simulink model "MLH2025"  (R2024b)
settings: Solver=VariableStepAuto  StartTime=0.0  StopTime=10.0  RelTol=1e-3
undefined symbols (not defined in the file): B, MPLX, Pi, PWM
settings Model: Creator=el2jo  LastModifiedBy=el2jo

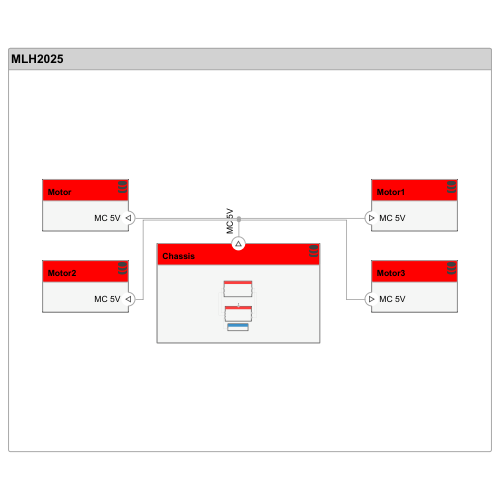
[thumbnail: Simulink's stored preview of the top-level diagram]
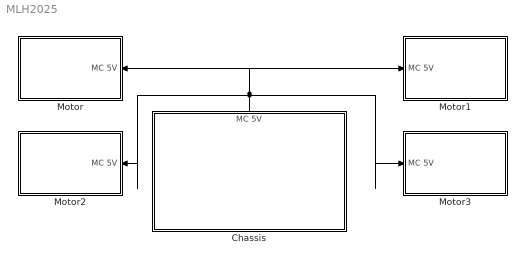
== system MLH2025 ==
  "Chassis " : Subsystem
      settings: PortSchema="{\"entries\":[{\"content\":{\"headerSize\":26,\"margin\":15,\"minimumSpacing\":25,\"sides\":[{\"content\":{},\"type\":\"ConnectorPlacement.EquallySpacedRectSide\",\"uuid\":\"9dc2c90c-aec4-43c7-8746-b592e26bfa16\"},{\"content\":{\"side\":\"RIGHT\"},\"type\":\"ConnectorPlacement.EquallySpacedRectSide\",\"uuid\":\"bdfb89bc-8823-48a4-99ae-46e8d46d5f72\"},{\"content\":{\"connectorIds\":[\"Out1\"],\"side\":\"TOP\"},\"type\":\"ConnectorPlacement.EquallySpacedRectSide\",\"uuid\":\"226bc484-5c65-4ece-8f5d-0589859e3e31\"}]},\"type\":\"ConnectorPlacement.EquallySpacedConnector\",\"uuid\":\"f9cc3cfe-bad8-451a-a9a4-a5a609f97b74\"}],\"packageUris\":[\"http://schema.mathworks.com/mf0/Connector/R2020b\"],\"version\":\"1.0\"}"
  Motor : Subsystem
      settings: PortSchema="{\"entries\":[{\"content\":{\"headerSize\":26,\"margin\":15,\"minimumSpacing\":25,\"sides\":[{\"content\":{},\"type\":\"ConnectorPlacement.EquallySpacedRectSide\",\"uuid\":\"9dc2c90c-aec4-43c7-8746-b592e26bfa16\"},{\"content\":{\"connectorIds\":[\"In1\"],\"side\":\"RIGHT\"},\"type\":\"ConnectorPlacement.EquallySpacedRectSide\",\"uuid\":\"bdfb89bc-8823-48a4-99ae-46e8d46d5f72\"},{\"content\":{\"side\":\"TOP\"},\"type\":\"ConnectorPlacement.EquallySpacedRectSide\",\"uuid\":\"226bc484-5c65-4ece-8f5d-0589859e3e31\"}]},\"type\":\"ConnectorPlacement.EquallySpacedConnector\",\"uuid\":\"f9cc3cfe-bad8-451a-a9a4-a5a609f97b74\"}],\"packageUris\":[\"http://schema.mathworks.com/mf0/Connector/R2020b\"],\"version\":\"1.0\"}"
  Motor1 : Subsystem
      settings: PortSchema="{\"entries\":[{\"content\":{\"headerSize\":26,\"margin\":15,\"minimumSpacing\":25,\"sides\":[{\"content\":{\"connectorIds\":[\"In1\"]},\"type\":\"ConnectorPlacement.EquallySpacedRectSide\",\"uuid\":\"9dc2c90c-aec4-43c7-8746-b592e26bfa16\"},{\"content\":{\"side\":\"RIGHT\"},\"type\":\"ConnectorPlacement.EquallySpacedRectSide\",\"uuid\":\"bdfb89bc-8823-48a4-99ae-46e8d46d5f72\"},{\"content\":{\"side\":\"TOP\"},\"type\":\"ConnectorPlacement.EquallySpacedRectSide\",\"uuid\":\"226bc484-5c65-4ece-8f5d-0589859e3e31\"}]},\"type\":\"ConnectorPlacement.EquallySpacedConnector\",\"uuid\":\"f9cc3cfe-bad8-451a-a9a4-a5a609f97b74\"}],\"packageUris\":[\"http://schema.mathworks.com/mf0/Connector/R2020b\"],\"version\":\"1.0\"}"
  Motor2 : Subsystem
      settings: PortSchema="{\"entries\":[{\"content\":{\"headerSize\":26,\"margin\":15,\"minimumSpacing\":25,\"sides\":[{\"content\":{},\"type\":\"ConnectorPlacement.EquallySpacedRectSide\",\"uuid\":\"9dc2c90c-aec4-43c7-8746-b592e26bfa16\"},{\"content\":{\"connectorIds\":[\"In1\"],\"side\":\"RIGHT\"},\"type\":\"ConnectorPlacement.EquallySpacedRectSide\",\"uuid\":\"bdfb89bc-8823-48a4-99ae-46e8d46d5f72\"},{\"content\":{\"side\":\"TOP\"},\"type\":\"ConnectorPlacement.EquallySpacedRectSide\",\"uuid\":\"226bc484-5c65-4ece-8f5d-0589859e3e31\"}]},\"type\":\"ConnectorPlacement.EquallySpacedConnector\",\"uuid\":\"f9cc3cfe-bad8-451a-a9a4-a5a609f97b74\"}],\"packageUris\":[\"http://schema.mathworks.com/mf0/Connector/R2020b\"],\"version\":\"1.0\"}"
  Motor3 : Subsystem
      settings: PortSchema="{\"entries\":[{\"content\":{\"headerSize\":26,\"margin\":15,\"minimumSpacing\":25,\"sides\":[{\"content\":{\"connectorIds\":[\"In1\"]},\"type\":\"ConnectorPlacement.EquallySpacedRectSide\",\"uuid\":\"9dc2c90c-aec4-43c7-8746-b592e26bfa16\"},{\"content\":{\"side\":\"RIGHT\"},\"type\":\"ConnectorPlacement.EquallySpacedRectSide\",\"uuid\":\"bdfb89bc-8823-48a4-99ae-46e8d46d5f72\"},{\"content\":{\"side\":\"TOP\"},\"type\":\"ConnectorPlacement.EquallySpacedRectSide\",\"uuid\":\"226bc484-5c65-4ece-8f5d-0589859e3e31\"}]},\"type\":\"ConnectorPlacement.EquallySpacedConnector\",\"uuid\":\"f9cc3cfe-bad8-451a-a9a4-a5a609f97b74\"}],\"packageUris\":[\"http://schema.mathworks.com/mf0/Connector/R2020b\"],\"version\":\"1.0\"}"
  wires:
  "Chassis "/1(MC 5V) -> Motor/1(MC 5V), Motor1/1(MC 5V), Motor3/1(MC 5V), Motor2/1(MC 5V)

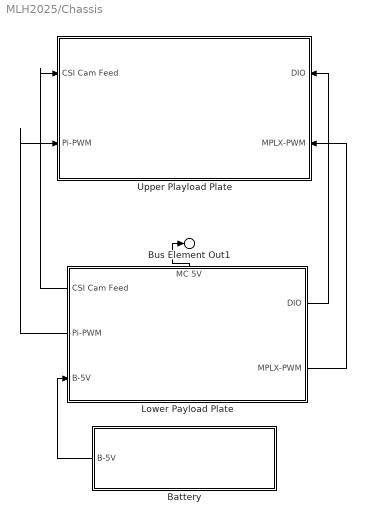
== system MLH2025/Chassis  ==
  Battery : Subsystem
      settings: PortSchema="{\"entries\":[{\"content\":{\"headerSize\":26,\"margin\":15,\"minimumSpacing\":25,\"sides\":[{\"content\":{\"connectorIds\":[\"Out1\"]},\"type\":\"ConnectorPlacement.EquallySpacedRectSide\",\"uuid\":\"9dc2c90c-aec4-43c7-8746-b592e26bfa16\"},{\"content\":{\"side\":\"RIGHT\"},\"type\":\"ConnectorPlacement.EquallySpacedRectSide\",\"uuid\":\"bdfb89bc-8823-48a4-99ae-46e8d46d5f72\"},{\"content\":{\"side\":\"TOP\"},\"type\":\"ConnectorPlacement.EquallySpacedRectSide\",\"uuid\":\"226bc484-5c65-4ece-8f5d-0589859e3e31\"}]},\"type\":\"ConnectorPlacement.EquallySpacedConnector\",\"uuid\":\"f9cc3cfe-bad8-451a-a9a4-a5a609f97b74\"}],\"packageUris\":[\"http://schema.mathworks.com/mf0/Connector/R2020b\"],\"version\":\"1.0\"}"
  Lower Payload Plate : Subsystem
      settings: PortSchema="{\"entries\":[{\"content\":{\"headerSize\":26,\"margin\":15,\"minimumSpacing\":25,\"sides\":[{\"content\":{\"connectorIds\":[\"Out1\",\"Out4\",\"In1\"]},\"type\":\"ConnectorPlacement.EquallySpacedRectSide\",\"uuid\":\"9dc2c90c-aec4-43c7-8746-b592e26bfa16\"},{\"content\":{\"connectorIds\":[\"Out3\",\"Out5\"],\"side\":\"RIGHT\"},\"type\":\"ConnectorPlacement.EquallySpacedRectSide\",\"uuid\":\"bdfb89bc-8823-48a4-99ae-46e8d46d5f72\"},{\"content\":{\"connectorIds\":[\"Out2\"],\"side\":\"TOP\"},\"type\":\"ConnectorPlacement.EquallySpacedRectSide\",\"uuid\":\"226bc484-5c65-4ece-8f5d-0589859e3e31\"}]},\"type\":\"ConnectorPlacement.EquallySpacedConnector\",\"uuid\":\"f9cc3cfe-bad8-451a-a9a4-a5a609f97b74\"}],\"packageUris\":[\"http://schema.mathworks.com/mf0/Connector/R2020b\"],\"version\":\"1.0\"}"
  Upper Playload Plate : Subsystem
      settings: PortSchema="{\"entries\":[{\"content\":{\"headerSize\":26,\"margin\":15,\"minimumSpacing\":25,\"sides\":[{\"content\":{\"connectorIds\":[\"In1\",\"In3\"]},\"type\":\"ConnectorPlacement.EquallySpacedRectSide\",\"uuid\":\"9dc2c90c-aec4-43c7-8746-b592e26bfa16\"},{\"content\":{\"connectorIds\":[\"In2\",\"In4\"],\"side\":\"RIGHT\"},\"type\":\"ConnectorPlacement.EquallySpacedRectSide\",\"uuid\":\"bdfb89bc-8823-48a4-99ae-46e8d46d5f72\"},{\"content\":{\"side\":\"TOP\"},\"type\":\"ConnectorPlacement.EquallySpacedRectSide\",\"uuid\":\"226bc484-5c65-4ece-8f5d-0589859e3e31\"}]},\"type\":\"ConnectorPlacement.EquallySpacedConnector\",\"uuid\":\"f9cc3cfe-bad8-451a-a9a4-a5a609f97b74\"}],\"packageUris\":[\"http://schema.mathworks.com/mf0/Connector/R2020b\"],\"version\":\"1.0\"}"
  Bus Element Out1 : Outport  PortName=MC 5V
  wires:
  Lower Payload Plate/5(MPLX-PWM) -> Upper Playload Plate/4(MPLX-PWM)
  Lower Payload Plate/4(Pi-PWM) -> Upper Playload Plate/3(Pi-PWM)
  Lower Payload Plate/3(DIO) -> Upper Playload Plate/2(DIO)
  Battery/1(B-5V) -> Lower Payload Plate/1(B-5V)
  Lower Payload Plate/2(MC 5V) -> Bus Element Out1/1
  Lower Payload Plate/1(CSI Cam Feed) -> Upper Playload Plate/1(CSI Cam Feed)

== system MLH2025/Motor ==
  Bus Element In1 : Inport  PortName=MC 5V

== system MLH2025/Motor1 ==
  Bus Element In1 : Inport  PortName=MC 5V

== system MLH2025/Motor2 ==
  Bus Element In1 : Inport  PortName=MC 5V

== system MLH2025/Motor3 ==
  Bus Element In1 : Inport  PortName=MC 5V

== system MLH2025/Chassis /Battery ==
  Bus Element Out1 : Outport  PortName=B-5V

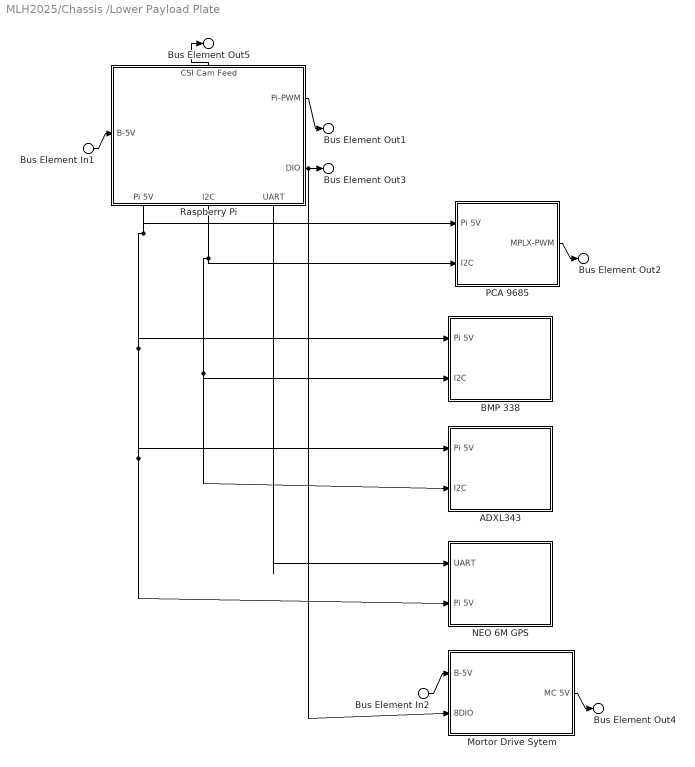
== system MLH2025/Chassis /Lower Payload Plate ==
  Bus Element In1 : Inport  PortName=B-5V
  Bus Element In2 : Inport  PortName=B-5V
  ADXL343 : Subsystem
      settings: PortSchema="{\"entries\":[{\"content\":{\"headerSize\":26,\"margin\":15,\"minimumSpacing\":25,\"sides\":[{\"content\":{\"connectorIds\":[\"In1\",\"In2\"]},\"type\":\"ConnectorPlacement.EquallySpacedRectSide\",\"uuid\":\"9dc2c90c-aec4-43c7-8746-b592e26bfa16\"},{\"content\":{\"side\":\"RIGHT\"},\"type\":\"ConnectorPlacement.EquallySpacedRectSide\",\"uuid\":\"bdfb89bc-8823-48a4-99ae-46e8d46d5f72\"},{\"content\":{\"side\":\"TOP\"},\"type\":\"ConnectorPlacement.EquallySpacedRectSide\",\"uuid\":\"226bc484-5c65-4ece-8f5d-0589859e3e31\"}]},\"type\":\"ConnectorPlacement.EquallySpacedConnector\",\"uuid\":\"f9cc3cfe-bad8-451a-a9a4-a5a609f97b74\"}],\"packageUris\":[\"http://schema.mathworks.com/mf0/Connector/R2020b\"],\"version\":\"1.0\"}"
  BMP 338 : Subsystem
      settings: PortSchema="{\"entries\":[{\"content\":{\"headerSize\":26,\"margin\":15,\"minimumSpacing\":25,\"sides\":[{\"content\":{\"connectorIds\":[\"In1\",\"In2\"]},\"type\":\"ConnectorPlacement.EquallySpacedRectSide\",\"uuid\":\"9dc2c90c-aec4-43c7-8746-b592e26bfa16\"},{\"content\":{\"side\":\"RIGHT\"},\"type\":\"ConnectorPlacement.EquallySpacedRectSide\",\"uuid\":\"bdfb89bc-8823-48a4-99ae-46e8d46d5f72\"},{\"content\":{\"side\":\"TOP\"},\"type\":\"ConnectorPlacement.EquallySpacedRectSide\",\"uuid\":\"226bc484-5c65-4ece-8f5d-0589859e3e31\"},{\"content\":{\"side\":\"BOTTOM\"},\"type\":\"ConnectorPlacement.EquallySpacedRectSide\",\"uuid\":\"99e16435-73fc-4f11-a495-18abe58af7ce\"}]},\"type\":\"ConnectorPlacement.EquallySpacedConnector\",\"uuid\":\"f9cc3cfe-bad8-451a-a9a4-a5a609f97b74\"}],\"packageUris\":[\"http://schema.mathworks.com/mf0/Connector/R2020b\"],\"version\":\"1.0\"}"
  Mortor Drive Sytem : Subsystem
      settings: PortSchema="{\"entries\":[{\"content\":{\"headerSize\":26,\"margin\":15,\"minimumSpacing\":25,\"sides\":[{\"content\":{\"connectorIds\":[\"In1\",\"In2\"]},\"type\":\"ConnectorPlacement.EquallySpacedRectSide\",\"uuid\":\"9dc2c90c-aec4-43c7-8746-b592e26bfa16\"},{\"content\":{\"connectorIds\":[\"Out1\"],\"side\":\"RIGHT\"},\"type\":\"ConnectorPlacement.EquallySpacedRectSide\",\"uuid\":\"bdfb89bc-8823-48a4-99ae-46e8d46d5f72\"},{\"content\":{\"side\":\"TOP\"},\"type\":\"ConnectorPlacement.EquallySpacedRectSide\",\"uuid\":\"226bc484-5c65-4ece-8f5d-0589859e3e31\"},{\"content\":{\"side\":\"BOTTOM\"},\"type\":\"ConnectorPlacement.EquallySpacedRectSide\",\"uuid\":\"135a2d99-9543-48c1-84f1-a8adb7010785\"}]},\"type\":\"ConnectorPlacement.EquallySpacedConnector\",\"uuid\":\"f9cc3cfe-bad8-451a-a9a4-a5a609f97b74\"}],\"packageUris\":[\"http://schema.mathworks.com/mf0/Connector/R2020b\"],\"version\":\"1.0\"}"
  NEO 6M GPS : Subsystem
      settings: PortSchema="{\"entries\":[{\"content\":{\"headerSize\":26,\"margin\":15,\"minimumSpacing\":25,\"sides\":[{\"content\":{\"connectorIds\":[\"In2\",\"In1\"]},\"type\":\"ConnectorPlacement.EquallySpacedRectSide\",\"uuid\":\"9dc2c90c-aec4-43c7-8746-b592e26bfa16\"},{\"content\":{\"side\":\"RIGHT\"},\"type\":\"ConnectorPlacement.EquallySpacedRectSide\",\"uuid\":\"bdfb89bc-8823-48a4-99ae-46e8d46d5f72\"},{\"content\":{\"side\":\"TOP\"},\"type\":\"ConnectorPlacement.EquallySpacedRectSide\",\"uuid\":\"226bc484-5c65-4ece-8f5d-0589859e3e31\"},{\"content\":{\"side\":\"BOTTOM\"},\"type\":\"ConnectorPlacement.EquallySpacedRectSide\",\"uuid\":\"07c50740-44ff-450e-bd99-694483ad2c77\"}]},\"type\":\"ConnectorPlacement.EquallySpacedConnector\",\"uuid\":\"f9cc3cfe-bad8-451a-a9a4-a5a609f97b74\"}],\"packageUris\":[\"http://schema.mathworks.com/mf0/Connector/R2020b\"],\"version\":\"1.0\"}"
  PCA 9685 : Subsystem
      settings: PortSchema="{\"entries\":[{\"content\":{\"headerSize\":26,\"margin\":15,\"minimumSpacing\":25,\"sides\":[{\"content\":{\"connectorIds\":[\"In1\",\"In2\"]},\"type\":\"ConnectorPlacement.EquallySpacedRectSide\",\"uuid\":\"9dc2c90c-aec4-43c7-8746-b592e26bfa16\"},{\"content\":{\"connectorIds\":[\"Out1\"],\"side\":\"RIGHT\"},\"type\":\"ConnectorPlacement.EquallySpacedRectSide\",\"uuid\":\"bdfb89bc-8823-48a4-99ae-46e8d46d5f72\"},{\"content\":{\"side\":\"TOP\"},\"type\":\"ConnectorPlacement.EquallySpacedRectSide\",\"uuid\":\"226bc484-5c65-4ece-8f5d-0589859e3e31\"}]},\"type\":\"ConnectorPlacement.EquallySpacedConnector\",\"uuid\":\"f9cc3cfe-bad8-451a-a9a4-a5a609f97b74\"}],\"packageUris\":[\"http://schema.mathworks.com/mf0/Connector/R2020b\"],\"version\":\"1.0\"}"
  "Raspberry Pi " : Subsystem
      settings: PortSchema="{\"entries\":[{\"content\":{\"headerSize\":26,\"margin\":15,\"minimumSpacing\":25,\"sides\":[{\"content\":{\"connectorIds\":[\"In1\"]},\"type\":\"ConnectorPlacement.EquallySpacedRectSide\",\"uuid\":\"9dc2c90c-aec4-43c7-8746-b592e26bfa16\"},{\"content\":{\"connectorIds\":[\"Out2\",\"Out3\"],\"side\":\"RIGHT\"},\"type\":\"ConnectorPlacement.EquallySpacedRectSide\",\"uuid\":\"bdfb89bc-8823-48a4-99ae-46e8d46d5f72\"},{\"content\":{\"connectorIds\":[\"Out1\"],\"side\":\"TOP\"},\"type\":\"ConnectorPlacement.EquallySpacedRectSide\",\"uuid\":\"226bc484-5c65-4ece-8f5d-0589859e3e31\"},{\"content\":{\"connectorIds\":[\"Out4\",\"Out5\",\"Out6\"],\"side\":\"BOTTOM\"},\"type\":\"ConnectorPlacement.EquallySpacedRectSide\",\"uuid\":\"e2d5389b-7d33-4c7a-8f47-39975d75565d\"}]},\"type\":\"ConnectorPlacement.EquallySpacedConnector\",\"uuid\":\"f9cc3cfe-bad8-451a-a9a4-a5a609f97b74\"}],\"packageUris\":[\"http://schema.mathworks.com/mf0/Connector/R2020b\"],\"version\":\"1.0\"}"
  Bus Element Out5 : Outport  PortName=CSI Cam Feed
  Bus Element Out4 : Outport  Port=2  PortName=MC 5V
  Bus Element Out3 : Outport  Port=3  PortName=DIO
  Bus Element Out1 : Outport  Port=4  PortName=Pi-PWM
  Bus Element Out2 : Outport  Port=5  PortName=MPLX-PWM
  wires:
  Bus Element In1/1 -> "Raspberry Pi "/1(B-5V)
  "Raspberry Pi "/2(Pi-PWM) -> Bus Element Out1/1
  "Raspberry Pi "/4("Pi 5V ") -> NEO 6M GPS/1("Pi 5V "), ADXL343/1("Pi 5V "), BMP 338/1("Pi 5V "), PCA 9685/1("Pi 5V ")
  Bus Element In2/1 -> Mortor Drive Sytem/1(B-5V)
  "Raspberry Pi "/5(I2C) -> BMP 338/2(I2C), ADXL343/2(I2C), PCA 9685/2(I2C)
  "Raspberry Pi "/6(UART) -> NEO 6M GPS/2(UART)
  "Raspberry Pi "/3(DIO) -> Mortor Drive Sytem/2(8DIO), Bus Element Out3/1
  "Raspberry Pi "/1(CSI Cam Feed) -> Bus Element Out5/1
  PCA 9685/1(MPLX-PWM) -> Bus Element Out2/1
  Mortor Drive Sytem/1(MC 5V) -> Bus Element Out4/1

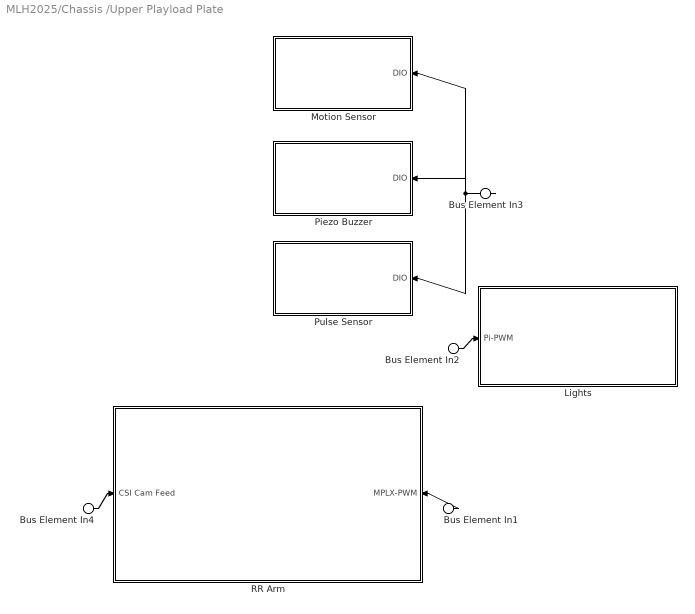
== system MLH2025/Chassis /Upper Playload Plate ==
  Bus Element In4 : Inport  PortName=CSI Cam Feed
  Bus Element In3 : Inport  Port=2  PortName=DIO
  Bus Element In2 : Inport  Port=3  PortName=Pi-PWM
  Bus Element In1 : Inport  Port=4  PortName=MPLX-PWM
  Lights : Subsystem
      settings: PortSchema="{\"entries\":[{\"content\":{\"headerSize\":26,\"margin\":15,\"minimumSpacing\":25,\"sides\":[{\"content\":{\"connectorIds\":[\"In1\"]},\"type\":\"ConnectorPlacement.EquallySpacedRectSide\",\"uuid\":\"9dc2c90c-aec4-43c7-8746-b592e26bfa16\"},{\"content\":{\"side\":\"RIGHT\"},\"type\":\"ConnectorPlacement.EquallySpacedRectSide\",\"uuid\":\"bdfb89bc-8823-48a4-99ae-46e8d46d5f72\"},{\"content\":{\"side\":\"TOP\"},\"type\":\"ConnectorPlacement.EquallySpacedRectSide\",\"uuid\":\"226bc484-5c65-4ece-8f5d-0589859e3e31\"}]},\"type\":\"ConnectorPlacement.EquallySpacedConnector\",\"uuid\":\"f9cc3cfe-bad8-451a-a9a4-a5a609f97b74\"}],\"packageUris\":[\"http://schema.mathworks.com/mf0/Connector/R2020b\"],\"version\":\"1.0\"}"
  Motion Sensor : Subsystem
      settings: PortSchema="{\"entries\":[{\"content\":{\"headerSize\":26,\"margin\":15,\"minimumSpacing\":25,\"sides\":[{\"content\":{},\"type\":\"ConnectorPlacement.EquallySpacedRectSide\",\"uuid\":\"9dc2c90c-aec4-43c7-8746-b592e26bfa16\"},{\"content\":{\"connectorIds\":[\"In1\"],\"side\":\"RIGHT\"},\"type\":\"ConnectorPlacement.EquallySpacedRectSide\",\"uuid\":\"bdfb89bc-8823-48a4-99ae-46e8d46d5f72\"},{\"content\":{\"side\":\"TOP\"},\"type\":\"ConnectorPlacement.EquallySpacedRectSide\",\"uuid\":\"226bc484-5c65-4ece-8f5d-0589859e3e31\"}]},\"type\":\"ConnectorPlacement.EquallySpacedConnector\",\"uuid\":\"f9cc3cfe-bad8-451a-a9a4-a5a609f97b74\"}],\"packageUris\":[\"http://schema.mathworks.com/mf0/Connector/R2020b\"],\"version\":\"1.0\"}"
  Piezo Buzzer : Subsystem
      settings: PortSchema="{\"entries\":[{\"content\":{\"headerSize\":26,\"margin\":15,\"minimumSpacing\":25,\"sides\":[{\"content\":{},\"type\":\"ConnectorPlacement.EquallySpacedRectSide\",\"uuid\":\"9dc2c90c-aec4-43c7-8746-b592e26bfa16\"},{\"content\":{\"connectorIds\":[\"In1\"],\"side\":\"RIGHT\"},\"type\":\"ConnectorPlacement.EquallySpacedRectSide\",\"uuid\":\"bdfb89bc-8823-48a4-99ae-46e8d46d5f72\"},{\"content\":{\"side\":\"TOP\"},\"type\":\"ConnectorPlacement.EquallySpacedRectSide\",\"uuid\":\"226bc484-5c65-4ece-8f5d-0589859e3e31\"}]},\"type\":\"ConnectorPlacement.EquallySpacedConnector\",\"uuid\":\"f9cc3cfe-bad8-451a-a9a4-a5a609f97b74\"}],\"packageUris\":[\"http://schema.mathworks.com/mf0/Connector/R2020b\"],\"version\":\"1.0\"}"
  Pulse Sensor : Subsystem
      settings: PortSchema="{\"entries\":[{\"content\":{\"headerSize\":26,\"margin\":15,\"minimumSpacing\":25,\"sides\":[{\"content\":{},\"type\":\"ConnectorPlacement.EquallySpacedRectSide\",\"uuid\":\"9dc2c90c-aec4-43c7-8746-b592e26bfa16\"},{\"content\":{\"connectorIds\":[\"In1\"],\"side\":\"RIGHT\"},\"type\":\"ConnectorPlacement.EquallySpacedRectSide\",\"uuid\":\"bdfb89bc-8823-48a4-99ae-46e8d46d5f72\"},{\"content\":{\"side\":\"TOP\"},\"type\":\"ConnectorPlacement.EquallySpacedRectSide\",\"uuid\":\"226bc484-5c65-4ece-8f5d-0589859e3e31\"}]},\"type\":\"ConnectorPlacement.EquallySpacedConnector\",\"uuid\":\"f9cc3cfe-bad8-451a-a9a4-a5a609f97b74\"}],\"packageUris\":[\"http://schema.mathworks.com/mf0/Connector/R2020b\"],\"version\":\"1.0\"}"
  "RR Arm " : Subsystem
      settings: PortSchema="{\"entries\":[{\"content\":{\"headerSize\":26,\"margin\":15,\"minimumSpacing\":25,\"sides\":[{\"content\":{\"connectorIds\":[\"In1\"]},\"type\":\"ConnectorPlacement.EquallySpacedRectSide\",\"uuid\":\"9dc2c90c-aec4-43c7-8746-b592e26bfa16\"},{\"content\":{\"connectorIds\":[\"In2\"],\"side\":\"RIGHT\"},\"type\":\"ConnectorPlacement.EquallySpacedRectSide\",\"uuid\":\"bdfb89bc-8823-48a4-99ae-46e8d46d5f72\"},{\"content\":{\"side\":\"TOP\"},\"type\":\"ConnectorPlacement.EquallySpacedRectSide\",\"uuid\":\"226bc484-5c65-4ece-8f5d-0589859e3e31\"}]},\"type\":\"ConnectorPlacement.EquallySpacedConnector\",\"uuid\":\"f9cc3cfe-bad8-451a-a9a4-a5a609f97b74\"}],\"packageUris\":[\"http://schema.mathworks.com/mf0/Connector/R2020b\"],\"version\":\"1.0\"}"
  wires:
  Bus Element In2/1 -> Lights/1(Pi-PWM)
  Bus Element In3/1 -> Piezo Buzzer/1(DIO), Pulse Sensor/1(DIO), Motion Sensor/1(DIO)
  Bus Element In1/1 -> "RR Arm "/2(MPLX-PWM)
  Bus Element In4/1 -> "RR Arm "/1(CSI Cam Feed)

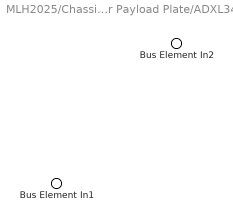
== system MLH2025/Chassis /Lower Payload Plate/ADXL343 ==
  Bus Element In2 : Inport  PortName=Pi 5V
  Bus Element In1 : Inport  Port=2  PortName=I2C

== system MLH2025/Chassis /Lower Payload Plate/BMP 338 ==
  Bus Element In2 : Inport  PortName=Pi 5V
  Bus Element In1 : Inport  Port=2  PortName=I2C

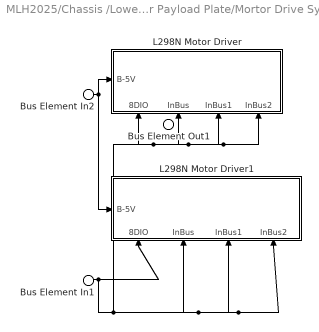
== system MLH2025/Chassis /Lower Payload Plate/Mortor Drive Sytem ==
  Bus Element In2 : Inport  PortName=B-5V
  Bus Element In1 : Inport  Port=2  PortName=8DIO
  L298N Motor Driver : Subsystem
      settings: PortSchema="{\"entries\":[{\"content\":{\"headerSize\":26,\"margin\":15,\"minimumSpacing\":25,\"sides\":[{\"content\":{\"connectorIds\":[\"In1\"]},\"type\":\"ConnectorPlacement.EquallySpacedRectSide\",\"uuid\":\"9dc2c90c-aec4-43c7-8746-b592e26bfa16\"},{\"content\":{\"side\":\"RIGHT\"},\"type\":\"ConnectorPlacement.EquallySpacedRectSide\",\"uuid\":\"bdfb89bc-8823-48a4-99ae-46e8d46d5f72\"},{\"content\":{\"side\":\"TOP\"},\"type\":\"ConnectorPlacement.EquallySpacedRectSide\",\"uuid\":\"226bc484-5c65-4ece-8f5d-0589859e3e31\"},{\"content\":{\"connectorIds\":[\"In2\",\"In3\",\"In4\",\"In5\"],\"side\":\"BOTTOM\"},\"type\":\"ConnectorPlacement.EquallySpacedRectSide\",\"uuid\":\"f688136e-6f14-4104-af2e-2d3d18e9ccdc\"}]},\"type\":\"ConnectorPlacement.EquallySpacedConnector\",\"uuid\":\"f9cc3cfe-bad8-451a-a9a4-a5a609f97b74\"}],\"packageUris\":[\"http://schema.mathworks.com/mf0/Connector/R2020b\"],\"version\":\"1.0\"}"
  L298N Motor Driver1 : Subsystem
      settings: PortSchema="{\"entries\":[{\"content\":{\"headerSize\":26,\"margin\":15,\"minimumSpacing\":25,\"sides\":[{\"content\":{\"connectorIds\":[\"In1\"]},\"type\":\"ConnectorPlacement.EquallySpacedRectSide\",\"uuid\":\"9dc2c90c-aec4-43c7-8746-b592e26bfa16\"},{\"content\":{\"side\":\"RIGHT\"},\"type\":\"ConnectorPlacement.EquallySpacedRectSide\",\"uuid\":\"bdfb89bc-8823-48a4-99ae-46e8d46d5f72\"},{\"content\":{\"side\":\"TOP\"},\"type\":\"ConnectorPlacement.EquallySpacedRectSide\",\"uuid\":\"226bc484-5c65-4ece-8f5d-0589859e3e31\"},{\"content\":{\"connectorIds\":[\"In2\",\"In3\",\"In4\",\"In5\"],\"side\":\"BOTTOM\"},\"type\":\"ConnectorPlacement.EquallySpacedRectSide\",\"uuid\":\"64243f08-7361-477c-b8cf-b33d7c02eba0\"}]},\"type\":\"ConnectorPlacement.EquallySpacedConnector\",\"uuid\":\"f9cc3cfe-bad8-451a-a9a4-a5a609f97b74\"}],\"packageUris\":[\"http://schema.mathworks.com/mf0/Connector/R2020b\"],\"version\":\"1.0\"}"
  Bus Element Out1 : Outport  PortName=MC 5V
  wires:
  Bus Element In1/1 -> L298N Motor Driver1/5(InBus2), L298N Motor Driver1/4(InBus1), L298N Motor Driver1/3(InBus), L298N Motor Driver/5(InBus2), L298N Motor Driver/4(InBus1), L298N Motor Driver/3(InBus), L298N Motor Driver/2(8DIO), L298N Motor Driver1/2(8DIO)
  Bus Element In2/1 -> L298N Motor Driver1/1(B-5V), L298N Motor Driver/1(B-5V)

== system MLH2025/Chassis /Lower Payload Plate/NEO 6M GPS ==
  Bus Element In2 : Inport  PortName=Pi 5V
  Bus Element In1 : Inport  Port=2  PortName=UART

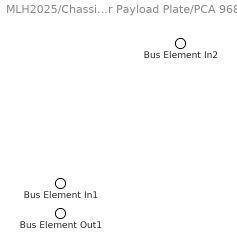
== system MLH2025/Chassis /Lower Payload Plate/PCA 9685 ==
  Bus Element In2 : Inport  PortName=Pi 5V
  Bus Element In1 : Inport  Port=2  PortName=I2C
  Bus Element Out1 : Outport  PortName=MPLX-PWM

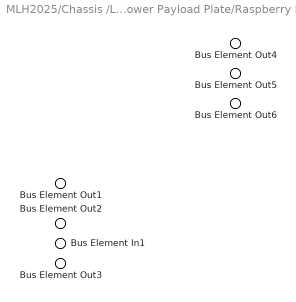
== system MLH2025/Chassis /Lower Payload Plate/Raspberry Pi  ==
  Bus Element In1 : Inport  PortName=B-5V
  Bus Element Out6 : Outport  PortName=CSI Cam Feed
  Bus Element Out5 : Outport  Port=2  PortName=Pi-PWM
  Bus Element Out4 : Outport  Port=3  PortName=DIO
  Bus Element Out1 : Outport  Port=4  PortName=Pi 5V
  Bus Element Out2 : Outport  Port=5  PortName=I2C
  Bus Element Out3 : Outport  Port=6  PortName=UART

== system MLH2025/Chassis /Upper Playload Plate/Lights ==
  Bus Element In1 : Inport  PortName=Pi-PWM

== system MLH2025/Chassis /Upper Playload Plate/Motion Sensor ==
  Bus Element In1 : Inport  PortName=DIO

== system MLH2025/Chassis /Upper Playload Plate/Piezo Buzzer ==
  Bus Element In1 : Inport  PortName=DIO

== system MLH2025/Chassis /Upper Playload Plate/Pulse Sensor ==
  Bus Element In1 : Inport  PortName=DIO

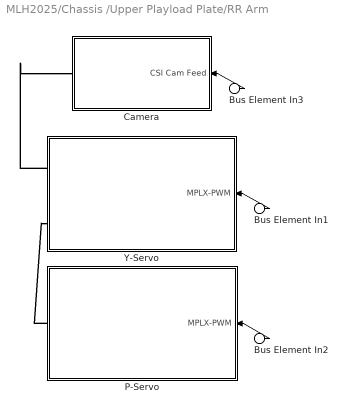
== system MLH2025/Chassis /Upper Playload Plate/RR Arm  ==
  Bus Element In3 : Inport  PortName=CSI Cam Feed
  Bus Element In1 : Inport  Port=2  PortName=MPLX-PWM
  Bus Element In2 : Inport  Port=2  PortName=MPLX-PWM
  Camera : Subsystem
      settings: PortSchema="{\"entries\":[{\"content\":{\"headerSize\":26,\"margin\":15,\"minimumSpacing\":25,\"sides\":[{\"content\":{\"connectorIds\":[\"LConn1\"]},\"type\":\"ConnectorPlacement.EquallySpacedRectSide\",\"uuid\":\"9dc2c90c-aec4-43c7-8746-b592e26bfa16\"},{\"content\":{\"connectorIds\":[\"In1\"],\"side\":\"RIGHT\"},\"type\":\"ConnectorPlacement.EquallySpacedRectSide\",\"uuid\":\"bdfb89bc-8823-48a4-99ae-46e8d46d5f72\"},{\"content\":{\"side\":\"TOP\"},\"type\":\"ConnectorPlacement.EquallySpacedRectSide\",\"uuid\":\"226bc484-5c65-4ece-8f5d-0589859e3e31\"}]},\"type\":\"ConnectorPlacement.EquallySpacedConnector\",\"uuid\":\"f9cc3cfe-bad8-451a-a9a4-a5a609f97b74\"}],\"packageUris\":[\"http://schema.mathworks.com/mf0/Connector/R2020b\"],\"version\":\"1.0\"}"
  "P-Servo " : Subsystem
      settings: PortSchema="{\"entries\":[{\"content\":{\"headerSize\":26,\"margin\":15,\"minimumSpacing\":25,\"sides\":[{\"content\":{\"connectorIds\":[\"LConn1\"]},\"type\":\"ConnectorPlacement.EquallySpacedRectSide\",\"uuid\":\"9dc2c90c-aec4-43c7-8746-b592e26bfa16\"},{\"content\":{\"connectorIds\":[\"In1\"],\"side\":\"RIGHT\"},\"type\":\"ConnectorPlacement.EquallySpacedRectSide\",\"uuid\":\"bdfb89bc-8823-48a4-99ae-46e8d46d5f72\"},{\"content\":{\"side\":\"TOP\"},\"type\":\"ConnectorPlacement.EquallySpacedRectSide\",\"uuid\":\"226bc484-5c65-4ece-8f5d-0589859e3e31\"}]},\"type\":\"ConnectorPlacement.EquallySpacedConnector\",\"uuid\":\"f9cc3cfe-bad8-451a-a9a4-a5a609f97b74\"}],\"packageUris\":[\"http://schema.mathworks.com/mf0/Connector/R2020b\"],\"version\":\"1.0\"}"
  Y-Servo : Subsystem
      settings: PortSchema="{\"entries\":[{\"content\":{\"headerSize\":26,\"margin\":15,\"minimumSpacing\":25,\"sides\":[{\"content\":{\"connectorIds\":[\"LConn1\",\"LConn2\"]},\"type\":\"ConnectorPlacement.EquallySpacedRectSide\",\"uuid\":\"9dc2c90c-aec4-43c7-8746-b592e26bfa16\"},{\"content\":{\"connectorIds\":[\"In1\"],\"side\":\"RIGHT\"},\"type\":\"ConnectorPlacement.EquallySpacedRectSide\",\"uuid\":\"bdfb89bc-8823-48a4-99ae-46e8d46d5f72\"},{\"content\":{\"side\":\"TOP\"},\"type\":\"ConnectorPlacement.EquallySpacedRectSide\",\"uuid\":\"226bc484-5c65-4ece-8f5d-0589859e3e31\"}]},\"type\":\"ConnectorPlacement.EquallySpacedConnector\",\"uuid\":\"f9cc3cfe-bad8-451a-a9a4-a5a609f97b74\"}],\"packageUris\":[\"http://schema.mathworks.com/mf0/Connector/R2020b\"],\"version\":\"1.0\"}"
  wires:
  Bus Element In1/1 -> Y-Servo/1(MPLX-PWM)
  Bus Element In2/1 -> "P-Servo "/1(MPLX-PWM)
  Bus Element In3/1 -> Camera/1(CSI Cam Feed)
  connections:
  "P-Servo "/LConn1 -- Y-Servo/LConn2
  Y-Servo/LConn1 -- Camera/LConn1

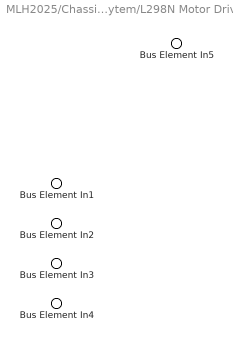
== system MLH2025/Chassis /Lower Payload Plate/Mortor Drive Sytem/L298N Motor Driver ==
  Bus Element In5 : Inport  PortName=B-5V
  Bus Element In1 : Inport  Port=2  PortName=8DIO
  Bus Element In2 : Inport  Port=3  PortName=InBus
  Bus Element In3 : Inport  Port=4  PortName=InBus1
  Bus Element In4 : Inport  Port=5  PortName=InBus2

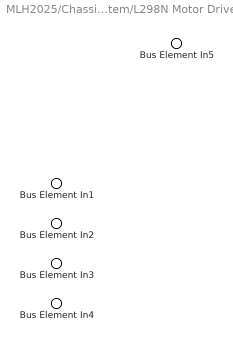
== system MLH2025/Chassis /Lower Payload Plate/Mortor Drive Sytem/L298N Motor Driver1 ==
  Bus Element In5 : Inport  PortName=B-5V
  Bus Element In1 : Inport  Port=2  PortName=8DIO
  Bus Element In2 : Inport  Port=3  PortName=InBus
  Bus Element In3 : Inport  Port=4  PortName=InBus1
  Bus Element In4 : Inport  Port=5  PortName=InBus2

== system MLH2025/Chassis /Upper Playload Plate/RR Arm /Camera ==
  Bus Element In1 : Inport  PortName=CSI Cam Feed
  Conn1 : PMIOPort  Side=Left

== system MLH2025/Chassis /Upper Playload Plate/RR Arm /P-Servo  ==
  Bus Element In1 : Inport  PortName=MPLX-PWM
  Conn1 : PMIOPort  Side=Left

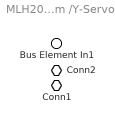
== system MLH2025/Chassis /Upper Playload Plate/RR Arm /Y-Servo ==
  Bus Element In1 : Inport  PortName=MPLX-PWM
  Conn2 : PMIOPort  Side=Left
  Conn1 : PMIOPort  Port=2  Side=Left
